simulink model "final_lock_in_fraser_FIR_sim"  (R2021a)
settings: Solver=FixedStepDiscrete  StartTime=0.0  StopTime=Inf  RelTol=1e-3  EnableMultiTasking=on
undefined symbols (not defined in the file): designMultirateFIR
libraries: dsparch4 x4, c2837xDlib x2, dspsrcs4 x2, dspmlti4 x2, c2802xlib x1
settings Model: SimulationMode=external  ExtModeBatchMode=on  ExtModeTrigDuration=8  Creator=Fraser Montandon  LastModifiedBy=Fraser Montandon
settings SolverCC: AutoInsertRateTranBlk=on
settings OptimizationCC: DefaultUnderspecifiedDataType=single  EnhancedBackFolding=on  PassReuseOutputArgsAs=Individual arguments  MaxStackSize=1024  OptimizeBlockOrder=speed  DifferentSizesBufferReuse=on  OptimizationCustomize=off  DenormalBehavior=FlushToZero  EfficientTunableParamExpr=on
settings DebuggingCC: ParameterTunabilityLossMsg=error
settings HardwareCC: ProdBitPerChar=16  ProdBitPerInt=16  ProdBitPerPointer=32  ProdBitPerSizeT=32  ProdBitPerPtrDiffT=32  ProdLargestAtomicInteger=Integer  ProdLargestAtomicFloat=None  ProdWordSize=16  ProdLongLongMode=on  ProdHWDeviceType=Texas Instruments->C2000
settings SFSimCC: MATLABDynamicMemAlloc=off
settings RTWCC: SystemTargetFile=ert.tlc  HardwareBoard=TI Delfino F28379D LaunchPad  TemplateMakefile=ert_default_tmf  Toolchain=Texas Instruments Code Composer Studio (C2000)  BuildConfiguration=Faster Runs
settings CodeAppCC: ForceParamTrailComments=on  IgnoreCustomStorageClasses=off  OperatorAnnotations=on  SimulinkDataObjDesc=on  SFDataObjDesc=on  InsertBlockDesc=on
settings ERTTargetCC: CodeReplacementLibrary=TI C28x  ExtModeTransport=3  ExtModeStaticAllocSize=10000

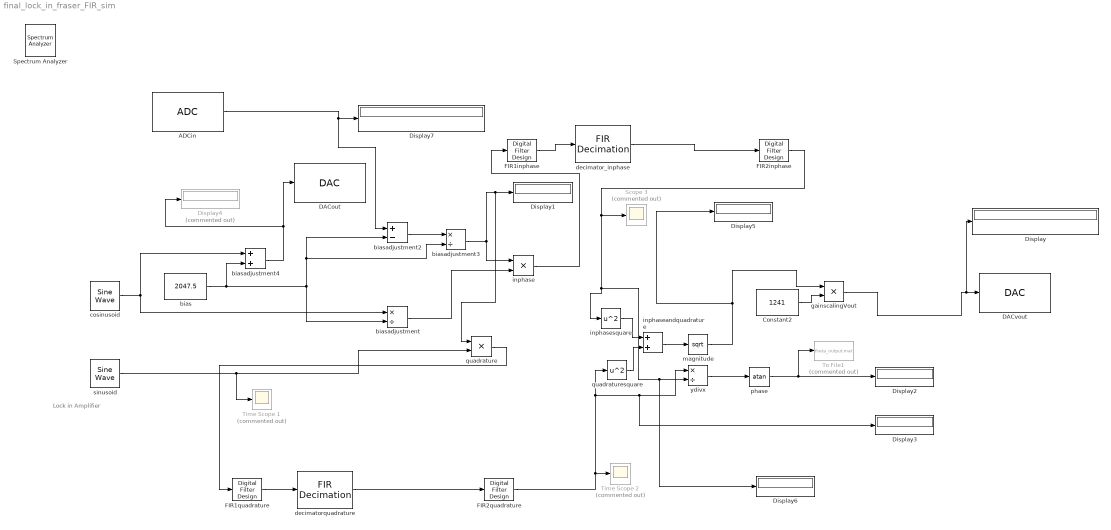
== system final_lock_in_fraser_FIR_sim ==
  note: Lock in Amplifier
  ADCin : c2802xlib/ADC  blkParamProc=C2000_Type4  ADCModule=A  samplingMode=Single sample mode  ADCResolution=12-bit (Single-ended input)  useSOC1=SOC0  useSOC2=SOC0_SOC1  SOCAcquisitionWindow=15  SOCTriggerSource=Software  SOCInterruptTrigger=No ADCINT  Ts=1/80000  dType=double  postInterrupt=off  interruptSel=ADCINT1  ADCINTContinuous=on  endma=off  chdma=1  conv1=ADCINA0  conv2=ADCINA0 and ADCINB0  conv1_Type4=ADCIN14  conv2_Type4=ADCIN0 and ADCIN1
  Constant2 : Constant  Value=1241
  DACout : c2837xDlib/DAC  channel=A  saturate=off
      settings: SourceProductBaseCode=TIC2000
  DACvout : c2837xDlib/DAC  channel=B  saturate=on
      settings: SourceProductBaseCode=TIC2000
  Display{,1..3,5..7} (7 alike) : Display
  Display4 : Display  Commented=on
  FIR1inphase : dsparch4/Digital Filter Design  mwdsp_browser_bugfix_var=off
  FIR1quadrature : dsparch4/Digital Filter Design  mwdsp_browser_bugfix_var=off
  FIR2inphase : dsparch4/Digital Filter Design  mwdsp_browser_bugfix_var=off
  FIR2quadrature : dsparch4/Digital Filter Design  mwdsp_browser_bugfix_var=off
  Scope 3 : Scope  Commented=on
  Time Scope 1 : Scope  Commented=on
      settings: Tag=Scope1
  Time Scope 2 : Scope  Commented=on
  To File1 : ToFile  Commented=on  Filename=theta_output.mat
      settings: Decimation=40000
  bias : Constant  Value=2047.5
  biasadjustment : Product  Inputs=*/
  biasadjustment2 : Sum  Inputs=+-
  biasadjustment3 : Product  Inputs=*/
  biasadjustment4 : Sum
  cosinusoid : dspsrcs4/Sine Wave  Amplitude=2047.5  Frequency=1000  Phase=pi/2  SampleMode=Discrete  OutComplex=Real  CompMethod=Table lookup  TableSize=Speed  SampleTime=1/80000  SamplesPerFrame=1  ResetState=Restart at time zero  OutputFrames=off  dataType=double  wordLen=16  udDataType=sfix(16)  fracBitsMode=Best precision  numFracBits=15  OutDataTypeStr=double  LastOutDataTypeStr=double
  decimator_inphase : dspmlti4/FIR Decimation  FilterSource=Auto  h=designMultirateFIR(1,2)  D=10  filtStruct=Direct form transposed  FilterObject=FDECIM  framing=Enforce single-rate processing  inputOffset=0  outputBufInitCond=0  roundingMode=Floor  overflowMode=off  firstCoeffDataTypeStr=Inherit: Same word length as input  firstCoeffMin=[]  firstCoeffMax=[]  firstCoeffLastDataTypeStr=Inherit: Same word length as input  outputDataTypeStr=Inherit: Same as accumulator  outputMin=[]  outputMax=[]  outputLastDataTypeStr=Inherit: Same as accumulator
  decimatorquadrature : dspmlti4/FIR Decimation  FilterSource=Auto  h=designMultirateFIR(1,2)  D=10  filtStruct=Direct form transposed  FilterObject=FDECIM  framing=Enforce single-rate processing  inputOffset=0  outputBufInitCond=0  roundingMode=Floor  overflowMode=off  firstCoeffDataTypeStr=Inherit: Same word length as input  firstCoeffMin=[]  firstCoeffMax=[]  firstCoeffLastDataTypeStr=Inherit: Same word length as input  outputDataTypeStr=Inherit: Same as accumulator  outputMin=[]  outputMax=[]  outputLastDataTypeStr=Inherit: Same as accumulator
  gainscalingVout : Product
  inphase : Product
  inphaseandquadrature : Sum
  inphasesquare : Math  Operator=square  SaturateOnIntegerOverflow=on
  magnitude : Sqrt  SaturateOnIntegerOverflow=on
  phase : Trigonometry  Operator=atan
  quadrature : Product
  quadraturesquare : Math  Operator=square  SaturateOnIntegerOverflow=on
  sinusoid : dspsrcs4/Sine Wave  Amplitude=1  Frequency=1000  Phase=0  SampleMode=Discrete  OutComplex=Real  CompMethod=Table lookup  TableSize=Speed  SampleTime=1/80000  SamplesPerFrame=1  ResetState=Restart at time zero  OutputFrames=off  dataType=double  wordLen=16  udDataType=sfix(16)  fracBitsMode=Best precision  numFracBits=15  OutDataTypeStr=double  LastOutDataTypeStr=double
  ydivx : Product  Inputs=*/
  Spectrum Analyzer : SpectrumAnalyzer  IOType=viewer
  wires:
  FIR2inphase/1 -> Display6/1, ydivx/2, inphasesquare/1, Scope 3/1
  magnitude/1 -> gainscalingVout/1, Display5/1
  biasadjustment/1 -> inphase/2
  bias/1 -> biasadjustment3/2, biasadjustment2/2, biasadjustment/2, biasadjustment4/2
  quadraturesquare/1 -> inphaseandquadrature/2
  cosinusoid/1 -> biasadjustment/1, biasadjustment4/1
  ydivx/1 -> phase/1
  sinusoid/1 -> quadrature/2, Time Scope 1/1
  inphaseandquadrature/1 -> magnitude/1
  biasadjustment3/1 -> Display1/1, quadrature/1, inphase/1
  inphasesquare/1 -> inphaseandquadrature/1
  biasadjustment4/1 -> Display4/1, DACout/1
  biasadjustment2/1 -> biasadjustment3/1
  FIR2quadrature/1 -> quadraturesquare/1, Display3/1, ydivx/1, Time Scope 2/1
  phase/1 -> Display2/1, To File1/1
  Constant2/1 -> gainscalingVout/2
  inphase/1 -> FIR1inphase/1
  ADCin/1 -> Display7/1, biasadjustment2/1
  gainscalingVout/1 -> Display/1, DACvout/1
  decimator_inphase/1 -> FIR2inphase/1
  quadrature/1 -> FIR1quadrature/1
  FIR1inphase/1 -> decimator_inphase/1
  FIR1quadrature/1 -> decimatorquadrature/1
  decimatorquadrature/1 -> FIR2quadrature/1
